simulink model "task4_model"  (R2021b)
settings: Solver=FixedStepAuto  StartTime=0.0  StopTime=50  FixedStep=0.0005  RelTol=1e-3
libraries: cstblocks x1
settings Model: Creator=den  LastModifiedBy=den

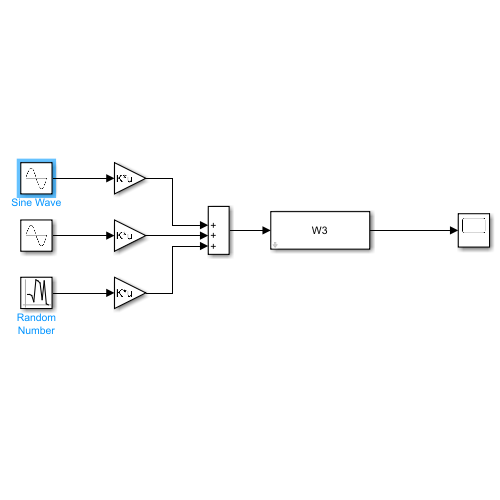
[thumbnail: Simulink's stored preview of the top-level diagram]
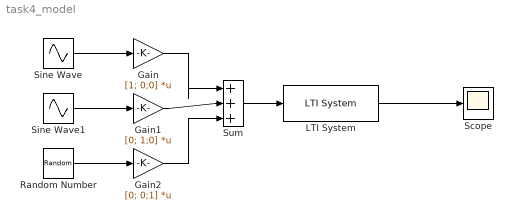
== system task4_model ==
  Gain : Gain  Gain=[1; 0;0]  Multiplication=Matrix(K*u)
  Gain1 : Gain  Gain=[0; 1;0]  Multiplication=Matrix(K*u)
  Gain2 : Gain  Gain=[0; 0;1]  Multiplication=Matrix(K*u)
  LTI System : cstblocks/LTI System  sys=W3  IC=[]
  Random Number : RandomNumber  Variance=2  Seed=1  SampleTime=0.1
  Scope : Scope
  Sine Wave : Sin  Amplitude=3  Bias=1/5  Frequency=2  Phase=-pi/3  SampleTime=0
  Sine Wave1 : Sin  Bias=-1/20  Frequency=2  Phase=(3*pi)/2  SampleTime=0
  Sum : Sum  Inputs=|+++
  wires:
  Sine Wave/1 -> Gain/1
  Gain/1 -> Sum/1
  LTI System/1 -> Scope/1
  Gain1/1 -> Sum/2
  Sum/1 -> LTI System/1
  Sine Wave1/1 -> Gain1/1
  Random Number/1 -> Gain2/1
  Gain2/1 -> Sum/3
